simulink model "EulerSim"  (R2023a)
settings: Solver=ode8  StartTime=0.0  StopTime=30  FixedStep=1e-3  RelTol=1e-3
values from neighbouring files (symbols this model uses):
  b = 0.1    [Eulerm.m]
  d = 0.1    [Eulerm.m]
  Im = 0.3    [Eulerm.m]
  J = 0.056    [Eulerm.m]
  Ke = 1.69    [Eulerm.m]
  Km = 1.69    [Eulerm.m]
  r = 1    [Eulerm.m]
  Rm = 2.2    [Eulerm.m]
libraries: slpidlib x2, shared6dof x1, simulink x1
settings Model: Creator=kutlukbilgearikan  LastModifiedBy=omert
settings SolverCC: AlgebraicLoopSolver=TrustRegion
settings DebuggingCC: UnconnectedInputMsg=warning  UnconnectedOutputMsg=warning  UnconnectedLineMsg=warning
settings ModelReferenceCC: EnableRefExpFcnMdlSchedulingChecks=on
settings RTWCC: DLArmComputeVersion=19.05

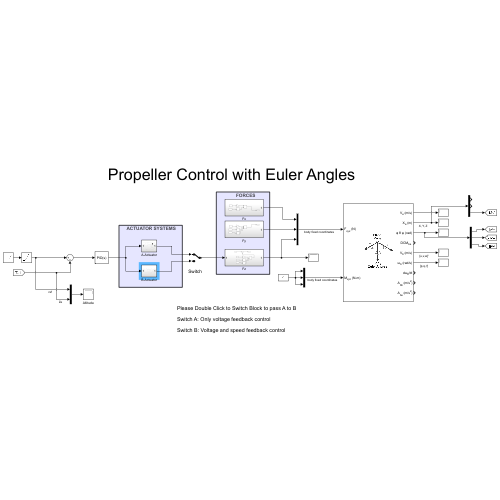
[thumbnail: Simulink's stored preview of the top-level diagram]
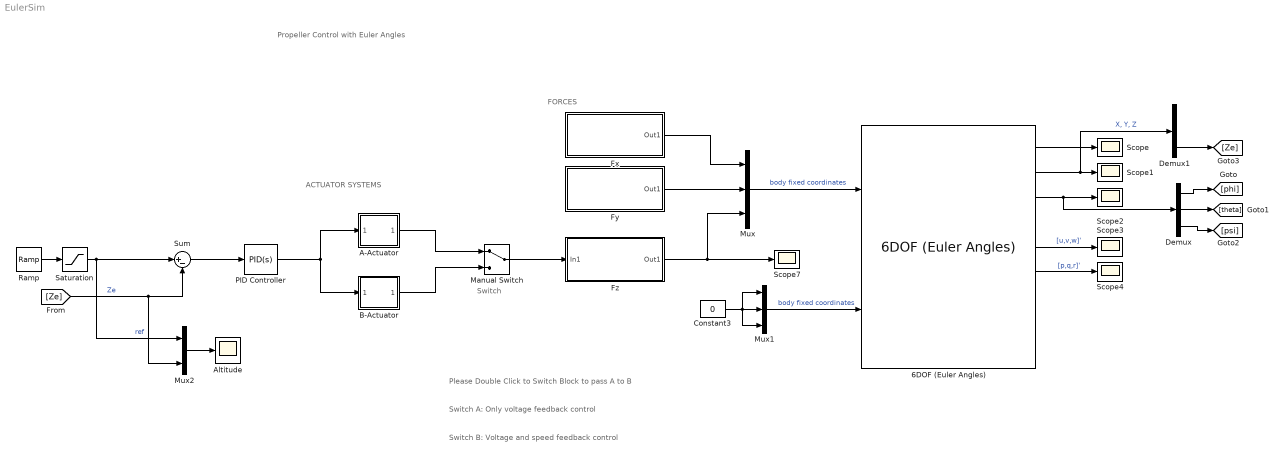
== system EulerSim ==
  note: Propeller Control with Euler Angles
  note: Please Double Click to Switch Block to pass A to B
  note: Switch
  note: ACTUATOR SYSTEMS
  note: FORCES
  note: Switch A: Only voltage feedback control
  note: Switch B: Voltage and speed feedback control
  6DOF (Euler Angles) : shared6dof/6DOF (Euler Angles)  units=Metric (MKS)  mtype=Fixed  rep=Euler Angles  xme_0=[0 0 0]  Vm_0=[0 0 0]  eul_0=[0 0 0]  pm_0=[0 0 0]  mass_0=3.8  mass_e=0.5  mass_f=2.0  inertia=0.01*eye(3)  inertia_e=eye(3)  inertia_f=2*eye(3)  k_quat=1.0  vre_flag=on  abi_flag=on  aMode=0  xme_statename=''  Vm_statename=''  eul_statename=''  quat_statename=''  pm_statename=''  mass_statename=''
  A-Actuator : Subsystem
  Altitude : Scope
  B-Actuator : Subsystem
  Constant3 : Constant  Value=0
  Demux : Demux  Outputs=3
  Demux1 : Demux  Outputs=3
  Fx : Subsystem
  Fy : Subsystem
  Fz : Subsystem
  Manual Switch : ManualSwitch
  Mux : Mux  Inputs=3
  Mux1 : Mux  Inputs=3
  Mux2 : Mux  Inputs=2
  PID Controller : slpidlib/PID Controller  Controller=PID  Form=Parallel  TimeDomain=Continuous-time  UseExternalTs=off  SampleTime=-1  IntegratorMethod=Forward Euler  FilterMethod=Forward Euler  ControllerParametersSource=internal  P=11  I=3  UseKiTs=off  D=5  N=1000  UseFilter=on  TunerSelectOption=Transfer Function Based (PID Tuner App)  InitialConditionSource=internal  InitialConditionForIntegrator=0  InitialConditionForFilter=0  DifferentiatorICPrevScaledInput=0  ExternalReset=none  TrackingMode=off  Kt=1  LimitOutput=off  SatLimitsSource=internal  UpperSaturationLimit=inf  LowerSaturationLimit=-inf  LinearizeAsGain=on  AntiWindupMode=none  Kb=1  LimitIntegrator=off  UpperIntegratorSaturationLimit=inf  LowerIntegratorSaturationLimit=-inf  POutMin=[]  POutMax=[]  IOutMin=[]  IOutMax=[]  DOutMin=[]  DOutMax=[]  NOutMin=[]  NOutMax=[]  SumOutMin=[]  SumOutMax=[]  SaturationOutMin=[]  SaturationOutMax=[]  PParamMin=[]  PParamMax=[]  IParamMin=[]  IParamMax=[]  DParamMin=[]  DParamMax=[]  NParamMin=[]  NParamMax=[]  KbParamMin=[]  KbParamMax=[]  KtParamMin=[]  KtParamMax=[]  KbOutMin=[]  KbOutMax=[]  KtOutMin=[]  KtOutMax=[]  IntegratorOutMin=[]  IntegratorOutMax=[]  FilterOutMin=[]  FilterOutMax=[]  SumI1OutMin=[]  SumI1OutMax=[]  SumI2OutMin=[]  SumI2OutMax=[]  SumI3OutMin=[]  SumI3OutMax=[]  SumI4OutMin=[]  SumI4OutMax=[]  SumDOutMin=[]  SumDOutMax=[]  DifferentiatorOutMin=[]  DifferentiatorOutMax=[]  FilterDiffOutCoefMin=[]  FilterDiffOutCoefMax=[]  ReciprocalOutMin=[]  ReciprocalOutMax=[]  SumDenOutMin=[]  SumDenOutMax=[]  SumNumOutMin=[]  SumNumOutMax=[]  DivideOutMin=[]  DivideOutMax=[]  UdiffTsProdOutMin=[]  UdiffTsProdOutMax=[]  NTsProdOutMin=[]  NTsProdOutMax=[]  UintegralTsProdOutMin=[]  UintegralTsProdOutMax=[]  UngainTsProdOutMin=[]  UngainTsProdOutMax=[]  ClampingZeroOutDataTypeStr=Inherit: Inherit via back propagation  ClampingZeroOutMin=[]  ClampingZeroOutMax=[]  FilterDenConstantOutDataTypeStr=Inherit: Inherit via back propagation  FilterDenConstantOutMin=[]  FilterDenConstantOutMax=[]  PCopyOutDataTypeStr=Inherit: Inherit via back propagation  PCopyOutMin=[]  PCopyOutMax=[]  NCopyOutDataTypeStr=Inherit: Inherit via back propagation  NCopyOutMin=[]  NCopyOutMax=[]  IntegratorContinuousStateAttributes=''  IntegratorStateMustResolveToSignalObject=off  IntegratorRTWStateStorageClass=Auto  FilterContinuousStateAttributes=''  FilterStateMustResolveToSignalObject=off  FilterRTWStateStorageClass=Auto  ParallelPVariant=InternalParameters  IdealPVariant=Disabled  IVariant=InternalParameters  DVariant=InternalParameters  IntegratorVariant=Continuous  SatVariant=Disabled  AWVariant=Passthrough  PCopyVariant=Disabled  TRVariant=Disabled  FdbkBlocksVariant=Forward  IdealPFdbkVariant=Disabled  SatFdbkVariant=Disabled  DerivativeFilterVariant=ContFilter  NVariant=InternalParameters  NCopyVariant=Disabled  FilterICVariant=InternalICsFilter  IntegratorICVariant=InternalICs  ExternalResetVariant=Disabled  TRSumVariant=Passthrough  SumFdbkVariant=Disabled  SumVariant=Sum_PID  TsampFilterVariant=InternalTs  TsampNgainVariant=Passthrough  TsampIntegralVariant=Disabled_SignalSpec  ExternalSaturationOutDataTypeStr=Inherit: Same as second input
  Ramp : simulink/Sources/Ramp  slope=-0.60  start=0  InitialOutput=0
  Saturation : Saturate  UpperLimit=0  LowerLimit=-5
  Scope{,1..4,7} (6 alike) : Scope
  Sum : Sum  Inputs=|+-
  wires:
  Mux/1 -> 6DOF (Euler Angles)/1  "body fixed coordinates"
  Mux1/1 -> 6DOF (Euler Angles)/2  "body fixed coordinates"
  Constant3/1 -> Mux1/2, Mux1/1, Mux1/3
  6DOF (Euler Angles)/1 -> Scope/1
  6DOF (Euler Angles)/2 -> Demux1/1, Scope1/1  "X, Y, Z"
  6DOF (Euler Angles)/3 -> Demux/1, Scope2/1
  6DOF (Euler Angles)/5 -> Scope3/1  "[u,v,w]'"
  6DOF (Euler Angles)/6 -> Scope4/1  "[p,q,r]'"
  Demux/1 -> [phi]
  Demux/2 -> [theta]
  Demux/3 -> [psi]
  Fx/1(Out1) -> Mux/1
  Fy/1(Out1) -> Mux/2
  Fz/1(Out1) -> Scope7/1, Mux/3
  Sum/1 -> PID Controller/1
  Ramp/1 -> Saturation/1
  Saturation/1 -> Mux2/1, Sum/1  "ref"
  Demux1/3 -> [Ze]
  [Ze] -> Mux2/2, Sum/2  "Ze"
  Mux2/1 -> Altitude/1
  PID Controller/1 -> A-Actuator/1(Input), B-Actuator/1(Input)
  A-Actuator/1(Out1) -> Manual Switch/1
  B-Actuator/1(Out1) -> Manual Switch/2
  Manual Switch/1 -> Fz/1(In1)

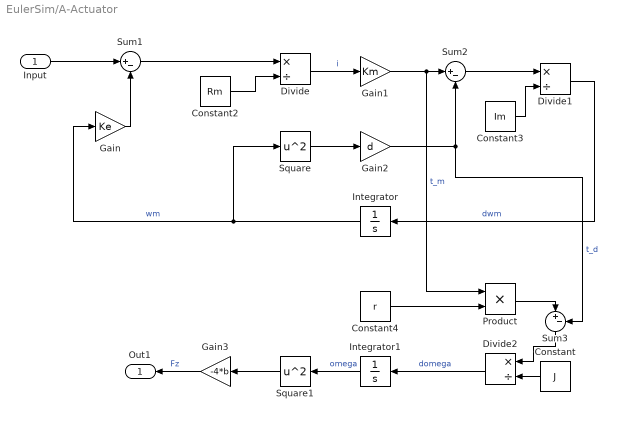
== system EulerSim/A-Actuator ==
  Input : Inport
  Constant : Constant  Value=J
  Constant2 : Constant  Value=Rm
  Constant3 : Constant  Value=Im
  Constant4 : Constant  Value=r
  Divide : Product  Inputs=*/
  Divide1 : Product  Inputs=*/
  Divide2 : Product  Inputs=*/
  Gain : Gain  Gain=Ke
  Gain1 : Gain  Gain=Km
  Gain2 : Gain  Gain=d
  Gain3 : Gain  Gain=-4*b
  Integrator : Integrator
  Integrator1 : Integrator
  Product : Product
  Square : Math  Operator=square
  Square1 : Math  Operator=square
  Sum1 : Sum  Inputs=|+-
  Sum2 : Sum  Inputs=|+-
  Sum3 : Sum  Inputs=|+-
  Out1 : Outport
  wires:
  Gain/1 -> Sum1/2
  Input/1 -> Sum1/1
  Sum1/1 -> Divide/1
  Constant2/1 -> Divide/2
  Divide/1 -> Gain1/1  "i"
  Gain1/1 -> Product/1, Sum2/1  "t_m"
  Integrator/1 -> Square/1, Gain/1  "wm"
  Square/1 -> Gain2/1
  Gain2/1 -> Sum3/2, Sum2/2  "t_d"
  Sum2/1 -> Divide1/1
  Constant3/1 -> Divide1/2
  Divide1/1 -> Integrator/1  "dwm"
  Constant4/1 -> Product/2
  Product/1 -> Sum3/1
  Sum3/1 -> Divide2/1
  Constant/1 -> Divide2/2
  Divide2/1 -> Integrator1/1  "domega"
  Integrator1/1 -> Square1/1  "omega"
  Square1/1 -> Gain3/1
  Gain3/1 -> Out1/1  "Fz"

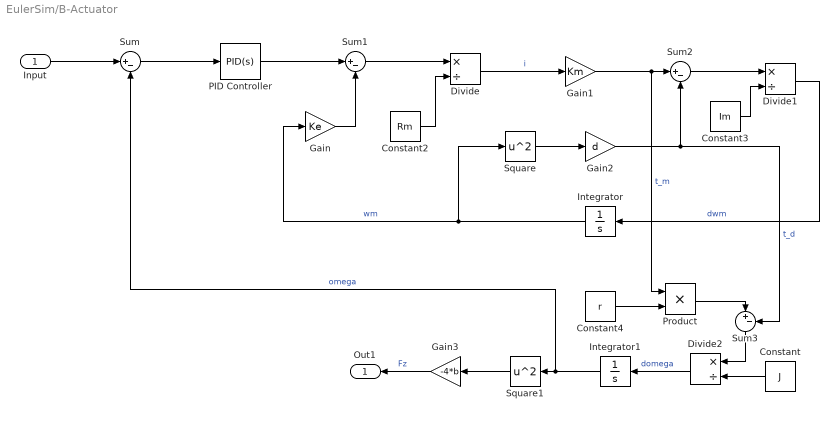
== system EulerSim/B-Actuator ==
  Input : Inport
  Constant : Constant  Value=J
  Constant2 : Constant  Value=Rm
  Constant3 : Constant  Value=Im
  Constant4 : Constant  Value=r
  Divide : Product  Inputs=*/
  Divide1 : Product  Inputs=*/
  Divide2 : Product  Inputs=*/
  Gain : Gain  Gain=Ke
  Gain1 : Gain  Gain=Km
  Gain2 : Gain  Gain=d
  Gain3 : Gain  Gain=-4*b
  Integrator : Integrator
  Integrator1 : Integrator
  PID Controller : slpidlib/PID Controller  Controller=PID  Form=Parallel  TimeDomain=Continuous-time  UseExternalTs=off  SampleTime=-1  IntegratorMethod=Forward Euler  FilterMethod=Forward Euler  ControllerParametersSource=internal  P=6.91821535673  I=4762.58547460805  UseKiTs=off  D=0.000745880968586172  N=1968.74689327737  UseFilter=on  TunerSelectOption=Transfer Function Based (PID Tuner App)  InitialConditionSource=internal  InitialConditionForIntegrator=0  InitialConditionForFilter=0  DifferentiatorICPrevScaledInput=0  ExternalReset=none  TrackingMode=off  Kt=1  LimitOutput=off  SatLimitsSource=internal  UpperSaturationLimit=inf  LowerSaturationLimit=-inf  LinearizeAsGain=on  AntiWindupMode=none  Kb=1  LimitIntegrator=off  UpperIntegratorSaturationLimit=inf  LowerIntegratorSaturationLimit=-inf  POutMin=[]  POutMax=[]  IOutMin=[]  IOutMax=[]  DOutMin=[]  DOutMax=[]  NOutMin=[]  NOutMax=[]  SumOutMin=[]  SumOutMax=[]  SaturationOutMin=[]  SaturationOutMax=[]  PParamMin=[]  PParamMax=[]  IParamMin=[]  IParamMax=[]  DParamMin=[]  DParamMax=[]  NParamMin=[]  NParamMax=[]  KbParamMin=[]  KbParamMax=[]  KtParamMin=[]  KtParamMax=[]  KbOutMin=[]  KbOutMax=[]  KtOutMin=[]  KtOutMax=[]  IntegratorOutMin=[]  IntegratorOutMax=[]  FilterOutMin=[]  FilterOutMax=[]  SumI1OutMin=[]  SumI1OutMax=[]  SumI2OutMin=[]  SumI2OutMax=[]  SumI3OutMin=[]  SumI3OutMax=[]  SumI4OutMin=[]  SumI4OutMax=[]  SumDOutMin=[]  SumDOutMax=[]  DifferentiatorOutMin=[]  DifferentiatorOutMax=[]  FilterDiffOutCoefMin=[]  FilterDiffOutCoefMax=[]  ReciprocalOutMin=[]  ReciprocalOutMax=[]  SumDenOutMin=[]  SumDenOutMax=[]  SumNumOutMin=[]  SumNumOutMax=[]  DivideOutMin=[]  DivideOutMax=[]  UdiffTsProdOutMin=[]  UdiffTsProdOutMax=[]  NTsProdOutMin=[]  NTsProdOutMax=[]  UintegralTsProdOutMin=[]  UintegralTsProdOutMax=[]  UngainTsProdOutMin=[]  UngainTsProdOutMax=[]  ClampingZeroOutDataTypeStr=Inherit: Inherit via back propagation  ClampingZeroOutMin=[]  ClampingZeroOutMax=[]  FilterDenConstantOutDataTypeStr=Inherit: Inherit via back propagation  FilterDenConstantOutMin=[]  FilterDenConstantOutMax=[]  PCopyOutDataTypeStr=Inherit: Inherit via back propagation  PCopyOutMin=[]  PCopyOutMax=[]  NCopyOutDataTypeStr=Inherit: Inherit via back propagation  NCopyOutMin=[]  NCopyOutMax=[]  IntegratorContinuousStateAttributes=''  IntegratorStateMustResolveToSignalObject=off  IntegratorRTWStateStorageClass=Auto  FilterContinuousStateAttributes=''  FilterStateMustResolveToSignalObject=off  FilterRTWStateStorageClass=Auto  ParallelPVariant=InternalParameters  IdealPVariant=Disabled  IVariant=InternalParameters  DVariant=InternalParameters  IntegratorVariant=Continuous  SatVariant=Disabled  AWVariant=Passthrough  PCopyVariant=Disabled  TRVariant=Disabled  FdbkBlocksVariant=Forward  IdealPFdbkVariant=Disabled  SatFdbkVariant=Disabled  DerivativeFilterVariant=ContFilter  NVariant=InternalParameters  NCopyVariant=Disabled  FilterICVariant=InternalICsFilter  IntegratorICVariant=InternalICs  ExternalResetVariant=Disabled  TRSumVariant=Passthrough  SumFdbkVariant=Disabled  SumVariant=Sum_PID  TsampFilterVariant=InternalTs  TsampNgainVariant=Passthrough  TsampIntegralVariant=Disabled_SignalSpec  ExternalSaturationOutDataTypeStr=Inherit: Same as second input
  Product : Product
  Square : Math  Operator=square
  Square1 : Math  Operator=square
  Sum{,1..3} (4 alike) : Sum  Inputs=|+-
  Out1 : Outport
  wires:
  Gain3/1 -> Out1/1  "Fz"
  Square1/1 -> Gain3/1
  Integrator1/1 -> Sum/2, Square1/1  "omega"
  Divide2/1 -> Integrator1/1  "domega"
  Constant/1 -> Divide2/2
  Sum3/1 -> Divide2/1
  Product/1 -> Sum3/1
  Constant4/1 -> Product/2
  Divide1/1 -> Integrator/1  "dwm"
  Constant3/1 -> Divide1/2
  Sum2/1 -> Divide1/1
  Gain2/1 -> Sum2/2, Sum3/2  "t_d"
  Square/1 -> Gain2/1
  Integrator/1 -> Square/1, Gain/1  "wm"
  Gain1/1 -> Sum2/1, Product/1  "t_m"
  Divide/1 -> Gain1/1  "i"
  Constant2/1 -> Divide/2
  Sum1/1 -> Divide/1
  Gain/1 -> Sum1/2
  Input/1 -> Sum/1
  Sum/1 -> PID Controller/1
  PID Controller/1 -> Sum1/1

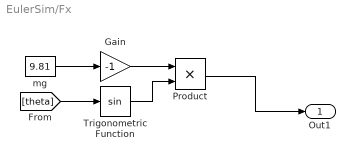
== system EulerSim/Fx ==
  Gain : Gain  Gain=-1
  Product : Product
  Trigonometric Function : Trigonometry
  mg : Constant  Value=9.81
  Out1 : Outport
  wires:
  Product/1 -> Out1/1
  mg/1 -> Gain/1
  [theta] -> Trigonometric Function/1
  Gain/1 -> Product/1
  Trigonometric Function/1 -> Product/2

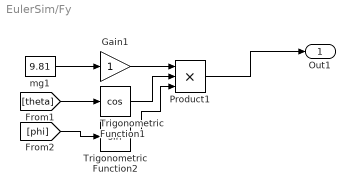
== system EulerSim/Fy ==
  Gain1 : Gain
  Product1 : Product  Inputs=3
  Trigonometric Function1 : Trigonometry  Operator=cos
  Trigonometric Function2 : Trigonometry
  mg1 : Constant  Value=9.81
  Out1 : Outport
  wires:
  Product1/1 -> Out1/1
  mg1/1 -> Gain1/1
  Trigonometric Function2/1 -> Product1/3
  Trigonometric Function1/1 -> Product1/2
  Gain1/1 -> Product1/1
  [phi] -> Trigonometric Function2/1
  [theta] -> Trigonometric Function1/1

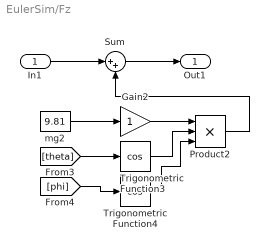
== system EulerSim/Fz ==
  In1 : Inport
  Gain2 : Gain
  Product2 : Product  Inputs=3
  Sum : Sum  Inputs=|++
  Trigonometric Function3 : Trigonometry  Operator=cos
  Trigonometric Function4 : Trigonometry  Operator=cos
  mg2 : Constant  Value=9.81
  Out1 : Outport
  wires:
  Trigonometric Function4/1 -> Product2/3
  mg2/1 -> Gain2/1
  Sum/1 -> Out1/1
  In1/1 -> Sum/1
  [theta] -> Trigonometric Function3/1
  Trigonometric Function3/1 -> Product2/2
  [phi] -> Trigonometric Function4/1
  Gain2/1 -> Product2/1
  Product2/1 -> Sum/2
